simulink model "test_parallel2"  (R2013a)
settings: Solver=ode45  StartTime=0.0  StopTime=inf  RelTol=1e-3
settings Model: Creator=michelr  LastModifiedBy=michelr

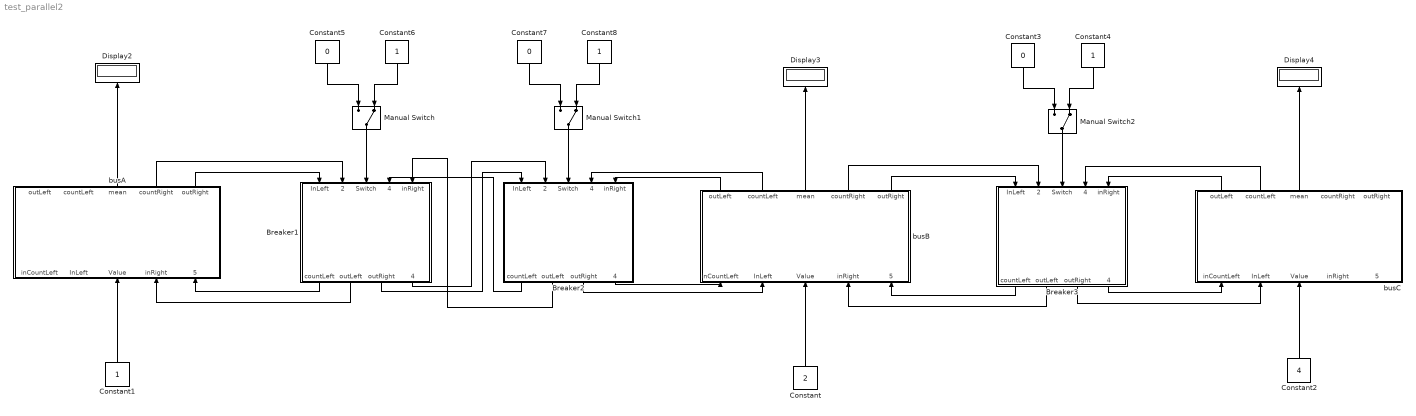
== system test_parallel2 ==
  Breaker1 : Subsystem
  Breaker2 : Subsystem
  Breaker3 : Subsystem
  Constant : Constant  Value=2
  Constant{1,4,6,8} (4 alike) : Constant
  Constant2 : Constant  Value=4
  Constant3 : Constant  Value=0
  Constant5 : Constant  Value=0
  Constant7 : Constant  Value=0
  Display2 : Display
  Display3 : Display
  Display4 : Display
  Manual Switch : ManualSwitch  CurrentSetting=0
  Manual Switch1 : ManualSwitch  CurrentSetting=0
  Manual Switch2 : ManualSwitch  CurrentSetting=0
  busA : Subsystem
  busB : Subsystem
  busC : Subsystem
  wires:
  busB/3(mean) -> Display3/1
  busA/3(mean) -> Display2/1
  busC/3(mean) -> Display4/1
  Constant1/1 -> busA/3(Value)
  Constant/1 -> busB/3(Value)
  Constant2/1 -> busC/3(Value)
  busA/5(outRight) -> Breaker1/1(InLeft)
  busA/4(countRight) -> Breaker1/2("inCountLeft ")
  Manual Switch/1 -> Breaker1/3("Switch ")
  Constant5/1 -> Manual Switch/1
  Constant6/1 -> Manual Switch/2
  Breaker1/1(countLeft) -> busA/5(inCountRight)
  Breaker1/2(outLeft) -> busA/4(inRight)
  Breaker1/3(outRight) -> Breaker2/1(InLeft)
  Breaker1/4(countRight) -> Breaker2/2("inCountLeft ")
  Breaker2/2(outLeft) -> Breaker1/5(inRight)
  Breaker2/1(countLeft) -> Breaker1/4(inCountRight)
  Constant7/1 -> Manual Switch1/1
  Constant8/1 -> Manual Switch1/2
  Manual Switch1/1 -> Breaker2/3("Switch ")
  busB/2(countLeft) -> Breaker2/4(inCountRight)
  busB/1(outLeft) -> Breaker2/5(inRight)
  Breaker2/3(outRight) -> busB/2(InLeft)
  Breaker2/4(countRight) -> busB/1("inCountLeft ")
  Constant3/1 -> Manual Switch2/1
  Constant4/1 -> Manual Switch2/2
  Manual Switch2/1 -> Breaker3/3("Switch ")
  busB/5(outRight) -> Breaker3/1(InLeft)
  busB/4(countRight) -> Breaker3/2("inCountLeft ")
  Breaker3/1(countLeft) -> busB/5(inCountRight)
  Breaker3/2(outLeft) -> busB/4(inRight)
  busC/1(outLeft) -> Breaker3/5(inRight)
  busC/2(countLeft) -> Breaker3/4(inCountRight)
  Breaker3/4(countRight) -> busC/1("inCountLeft ")
  Breaker3/3(outRight) -> busC/2(InLeft)

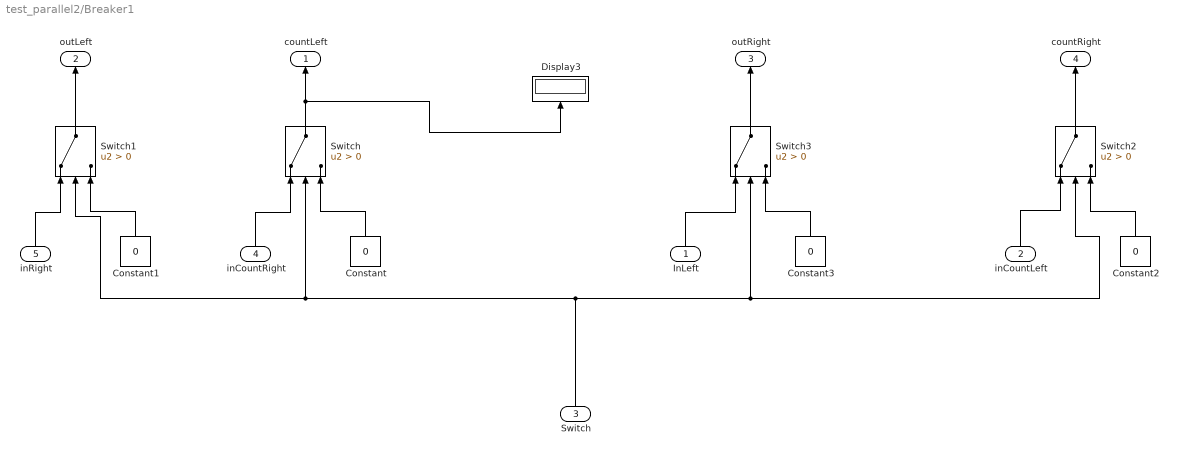
== system test_parallel2/Breaker1 ==
  InLeft : Inport
  "inCountLeft " : Inport  Port=2
  "Switch " : Inport  Port=3
  inCountRight : Inport  Port=4
  inRight : Inport  Port=5
  Constant{,1..3} (4 alike) : Constant  Value=0
  Display3 : Display
  Switch{,1..3} (4 alike) : Switch  Criteria=u2 > Threshold
  countLeft : Outport
  outLeft : Outport  Port=2
  outRight : Outport  Port=3
  countRight : Outport  Port=4
  wires:
  "Switch "/1 -> Switch2/2, Switch3/2, Switch1/2, Switch/2
  inCountRight/1 -> Switch/1
  Switch/1 -> Display3/1, countLeft/1
  Constant/1 -> Switch/3
  Constant1/1 -> Switch1/3
  inRight/1 -> Switch1/1
  Switch1/1 -> outLeft/1
  Constant2/1 -> Switch2/3
  Constant3/1 -> Switch3/3
  InLeft/1 -> Switch3/1
  Switch3/1 -> outRight/1
  Switch2/1 -> countRight/1
  "inCountLeft "/1 -> Switch2/1

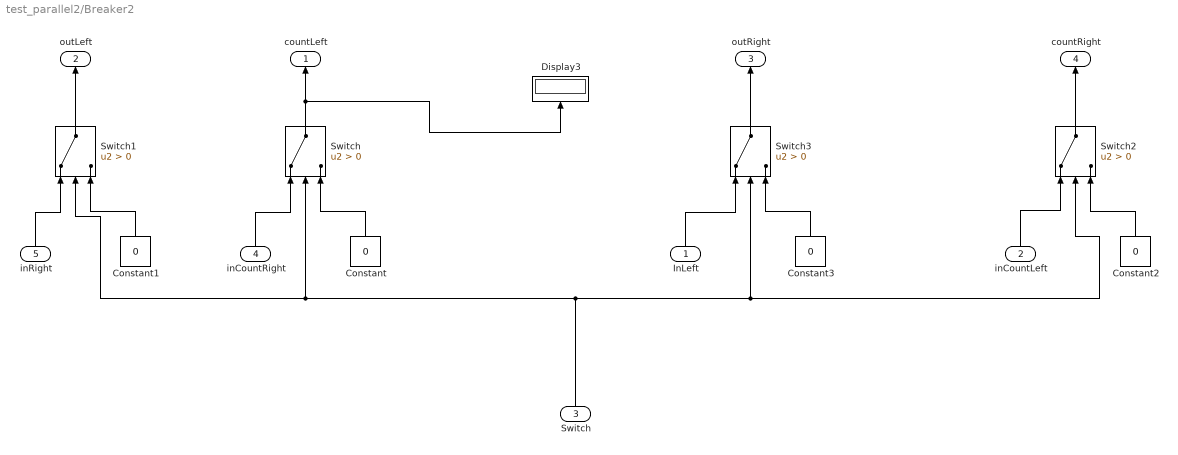
== system test_parallel2/Breaker2 ==
  InLeft : Inport
  "inCountLeft " : Inport  Port=2
  "Switch " : Inport  Port=3
  inCountRight : Inport  Port=4
  inRight : Inport  Port=5
  Constant{,1..3} (4 alike) : Constant  Value=0
  Display3 : Display
  Switch{,1..3} (4 alike) : Switch  Criteria=u2 > Threshold
  countLeft : Outport
  outLeft : Outport  Port=2
  outRight : Outport  Port=3
  countRight : Outport  Port=4
  wires:
  "Switch "/1 -> Switch2/2, Switch3/2, Switch1/2, Switch/2
  inCountRight/1 -> Switch/1
  Switch/1 -> Display3/1, countLeft/1
  Constant/1 -> Switch/3
  Constant1/1 -> Switch1/3
  inRight/1 -> Switch1/1
  Switch1/1 -> outLeft/1
  Constant2/1 -> Switch2/3
  Constant3/1 -> Switch3/3
  InLeft/1 -> Switch3/1
  Switch3/1 -> outRight/1
  Switch2/1 -> countRight/1
  "inCountLeft "/1 -> Switch2/1

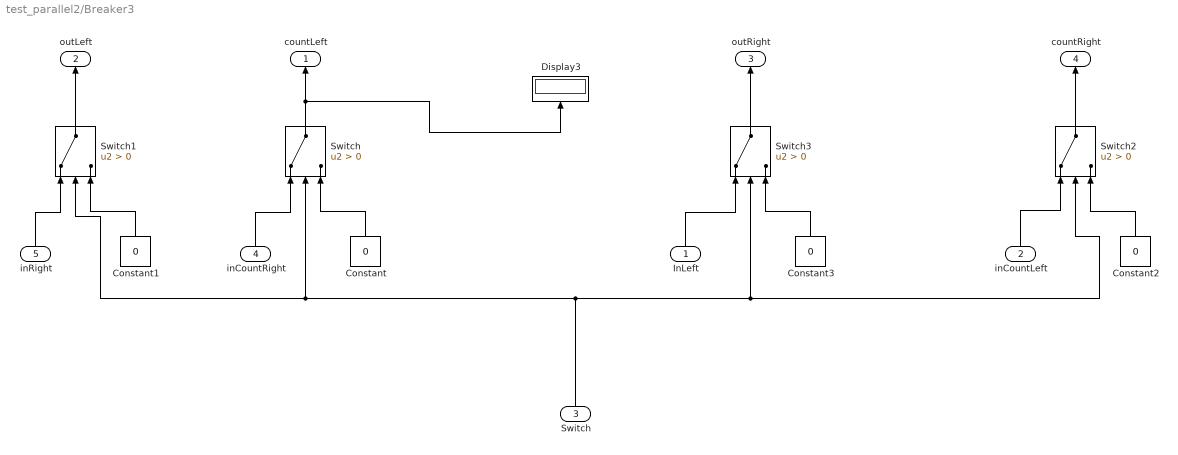
== system test_parallel2/Breaker3 ==
  InLeft : Inport
  "inCountLeft " : Inport  Port=2
  "Switch " : Inport  Port=3
  inCountRight : Inport  Port=4
  inRight : Inport  Port=5
  Constant{,1..3} (4 alike) : Constant  Value=0
  Display3 : Display
  Switch{,1..3} (4 alike) : Switch  Criteria=u2 > Threshold
  countLeft : Outport
  outLeft : Outport  Port=2
  outRight : Outport  Port=3
  countRight : Outport  Port=4
  wires:
  "Switch "/1 -> Switch2/2, Switch3/2, Switch1/2, Switch/2
  inCountRight/1 -> Switch/1
  Switch/1 -> Display3/1, countLeft/1
  Constant/1 -> Switch/3
  Constant1/1 -> Switch1/3
  inRight/1 -> Switch1/1
  Switch1/1 -> outLeft/1
  Constant2/1 -> Switch2/3
  Constant3/1 -> Switch3/3
  InLeft/1 -> Switch3/1
  Switch3/1 -> outRight/1
  Switch2/1 -> countRight/1
  "inCountLeft "/1 -> Switch2/1

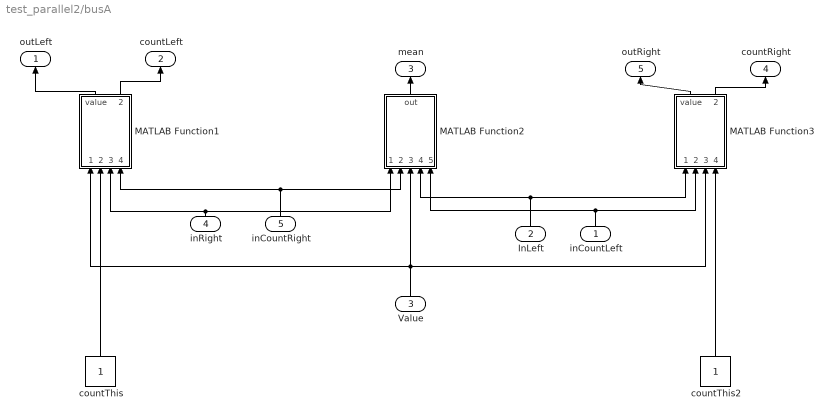
== system test_parallel2/busA ==
  "inCountLeft " : Inport
  InLeft : Inport  Port=2
  Value : Inport  Port=3
  inRight : Inport  Port=4
  inCountRight : Inport  Port=5
  MATLAB Function1 : MATLAB Function  TreatAsAtomicUnit=on
  MATLAB Function2 : MATLAB Function  TreatAsAtomicUnit=on
  MATLAB Function3 : MATLAB Function  TreatAsAtomicUnit=on
  countThis : Constant
  countThis2 : Constant
  outLeft : Outport
  countLeft : Outport  Port=2
  mean : Outport  Port=3
  countRight : Outport  Port=4
  outRight : Outport  Port=5
  wires:
  MATLAB Function3/1(value) -> outRight/1
  MATLAB Function2/1(out) -> mean/1
  MATLAB Function1/2(count) -> countLeft/1
  MATLAB Function1/1(value) -> outLeft/1
  MATLAB Function3/2(count) -> countRight/1
  InLeft/1 -> MATLAB Function3/1(in1), MATLAB Function2/4(in3)
  "inCountLeft "/1 -> MATLAB Function2/5(number3), MATLAB Function3/2(count1)
  inRight/1 -> MATLAB Function2/1(in1), MATLAB Function1/3(in2)
  inCountRight/1 -> MATLAB Function1/4(count2), MATLAB Function2/2(number1)
  Value/1 -> MATLAB Function3/3(in2), MATLAB Function1/1(in1), MATLAB Function2/3(in2)
  countThis2/1 -> MATLAB Function3/4(count2)
  countThis/1 -> MATLAB Function1/2(count1)

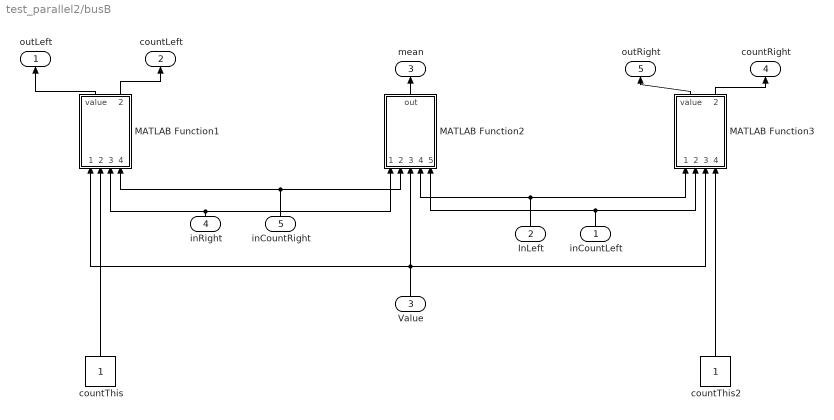
== system test_parallel2/busB ==
  "inCountLeft " : Inport
  InLeft : Inport  Port=2
  Value : Inport  Port=3
  inRight : Inport  Port=4
  inCountRight : Inport  Port=5
  MATLAB Function1 : MATLAB Function  TreatAsAtomicUnit=on
  MATLAB Function2 : MATLAB Function  TreatAsAtomicUnit=on
  MATLAB Function3 : MATLAB Function  TreatAsAtomicUnit=on
  countThis : Constant
  countThis2 : Constant
  outLeft : Outport
  countLeft : Outport  Port=2
  mean : Outport  Port=3
  countRight : Outport  Port=4
  outRight : Outport  Port=5
  wires:
  MATLAB Function3/1(value) -> outRight/1
  MATLAB Function2/1(out) -> mean/1
  MATLAB Function1/2(count) -> countLeft/1
  MATLAB Function1/1(value) -> outLeft/1
  MATLAB Function3/2(count) -> countRight/1
  InLeft/1 -> MATLAB Function2/4(in3), MATLAB Function3/1(in1)
  "inCountLeft "/1 -> MATLAB Function3/2(count1), MATLAB Function2/5(number3)
  inRight/1 -> MATLAB Function2/1(in1), MATLAB Function1/3(in2)
  inCountRight/1 -> MATLAB Function2/2(number1), MATLAB Function1/4(count2)
  Value/1 -> MATLAB Function2/3(in2), MATLAB Function3/3(in2), MATLAB Function1/1(in1)
  countThis2/1 -> MATLAB Function3/4(count2)
  countThis/1 -> MATLAB Function1/2(count1)

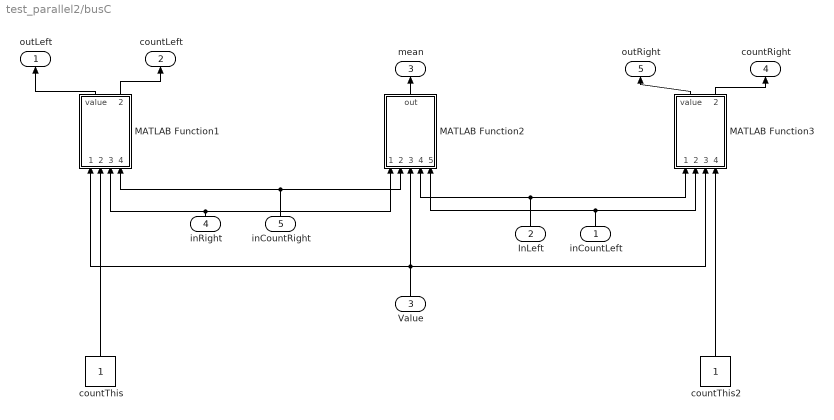
== system test_parallel2/busC ==
  "inCountLeft " : Inport
  InLeft : Inport  Port=2
  Value : Inport  Port=3
  inRight : Inport  Port=4
  inCountRight : Inport  Port=5
  MATLAB Function1 : MATLAB Function  TreatAsAtomicUnit=on
  MATLAB Function2 : MATLAB Function  TreatAsAtomicUnit=on
  MATLAB Function3 : MATLAB Function  TreatAsAtomicUnit=on
  countThis : Constant
  countThis2 : Constant
  outLeft : Outport
  countLeft : Outport  Port=2
  mean : Outport  Port=3
  countRight : Outport  Port=4
  outRight : Outport  Port=5
  wires:
  MATLAB Function3/2(count) -> countRight/1
  MATLAB Function1/1(value) -> outLeft/1
  MATLAB Function1/2(count) -> countLeft/1
  MATLAB Function2/1(out) -> mean/1
  MATLAB Function3/1(value) -> outRight/1
  InLeft/1 -> MATLAB Function3/1(in1), MATLAB Function2/4(in3)
  "inCountLeft "/1 -> MATLAB Function2/5(number3), MATLAB Function3/2(count1)
  inRight/1 -> MATLAB Function2/1(in1), MATLAB Function1/3(in2)
  inCountRight/1 -> MATLAB Function1/4(count2), MATLAB Function2/2(number1)
  Value/1 -> MATLAB Function3/3(in2), MATLAB Function1/1(in1), MATLAB Function2/3(in2)
  countThis2/1 -> MATLAB Function3/4(count2)
  countThis/1 -> MATLAB Function1/2(count1)

== matlab function test_parallel2/busB/MATLAB Function1 ==
  data: in1 input; count1 input; value output; in2 input; count2 input; count output
function [value,count] = fcn(in1,count1,in2,count2)
count = 0;
value = 0;
if count1 > 0
    count = count + count1;
    value = value + in1;
end
    
if count2 > 0
    count = count + count2;
    value = value + in2;
end

end

== matlab function test_parallel2/busB/MATLAB Function3 ==
  data: in1 input; count1 input; value output; in2 input; count2 input; count output
function [value,count] = fcn(in1,count1,in2,count2)
count = 0;
value = 0;
if count1 > 0
    count = count + count1;
    value = value + in1;
end
    
if count2 > 0
    count = count + count2;
    value = value + in2;
end

end

== matlab function test_parallel2/busB/MATLAB Function2 ==
  data: in1 input; number1 input; out output; in2 input; in3 input; number3 input
function out  = fcn(in1,number1,in2,in3,number3)
count = 1;
out = in2;

if number1 > 0
    out = out + in1;
    count = count + number1;
end
if number3 > 0
    out = out + in3;
    count = count + number3;
end

out = out / count;
end

== matlab function test_parallel2/busC/MATLAB Function1 ==
  data: in1 input; count1 input; value output; in2 input; count2 input; count output
function [value,count] = fcn(in1,count1,in2,count2)
count = 0;
value = 0;
if count1 > 0
    count = count + count1;
    value = value + in1;
end
    
if count2 > 0
    count = count + count2;
    value = value + in2;
end

end

== matlab function test_parallel2/busC/MATLAB Function2 ==
  data: in1 input; number1 input; out output; in2 input; in3 input; number3 input
function out  = fcn(in1,number1,in2,in3,number3)
count = 1;
out = in2;

if number1 > 0
    out = out + in1;
    count = count + number1;
end
if number3 > 0
    out = out + in3;
    count = count + number3;
end

out = out / count;
end

== matlab function test_parallel2/busC/MATLAB Function3 ==
  data: in1 input; count1 input; value output; in2 input; count2 input; count output
function [value,count] = fcn(in1,count1,in2,count2)
count = 0;
value = 0;
if count1 > 0
    count = count + count1;
    value = value + in1;
end
    
if count2 > 0
    count = count + count2;
    value = value + in2;
end

end

== matlab function test_parallel2/busA/MATLAB Function1 ==
  data: in1 input; count1 input; value output; in2 input; count2 input; count output
function [value,count] = fcn(in1,count1,in2,count2)
count = 0;
value = 0;
if count1 > 0
    count = count + count1;
    value = value + in1;
end
    
if count2 > 0
    count = count + count2;
    value = value + in2;
end

end

== matlab function test_parallel2/busA/MATLAB Function2 ==
  data: in1 input; number1 input; out output; in2 input; in3 input; number3 input
function out  = fcn(in1,number1,in2,in3,number3)
count = 1;
out = in2;

if number1 > 0
    out = out + in1;
    count = count + number1;
end
if number3 > 0
    out = out + in3;
    count = count + number3;
end

out = out / count;
end

== matlab function test_parallel2/busA/MATLAB Function3 ==
  data: in1 input; count1 input; value output; in2 input; count2 input; count output
function [value,count] = fcn(in1,count1,in2,count2)
count = 0;
value = 0;
if count1 > 0
    count = count + count1;
    value = value + in1;
end
    
if count2 > 0
    count = count + count2;
    value = value + in2;
end

end
